simulink model "si5c_bouncing_ball_inelastic"  (R2024a)
settings: Solver=VariableStepAuto  StartTime=0.0  StopTime=10  RelTol=1e-3
values from neighbouring files (symbols this model uses):
  c = 1    [sim21_solution.m]
undefined symbols (not defined in the file or in its folder): g, h
settings Model: Creator=ocean  LastModifiedBy=ocean

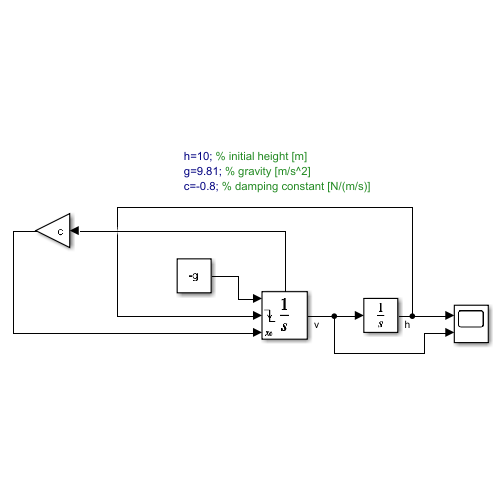
[thumbnail: Simulink's stored preview of the top-level diagram]
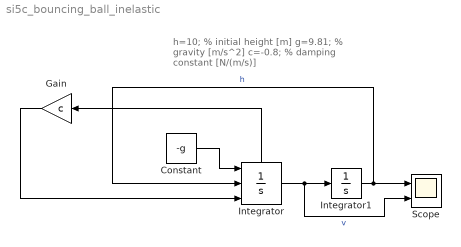
== system si5c_bouncing_ball_inelastic ==
  note: h=10; % initial height [m]
      | g=9.81; % gravity [m/s^2]
      | c=-0.8; % damping constant [N/(m/s)]
  Constant : Constant  Value=-g
  Gain : Gain  Gain=c
  Integrator : Integrator  ExternalReset=falling  InitialConditionSource=external  ShowStatePort=on
  Integrator1 : Integrator  InitialCondition=h
  Scope : Scope  NumInputPorts=2
  wires:
  Integrator/1 -> Scope/2, Integrator1/1  "v"
  Constant/1 -> Integrator/1
  Integrator1/1 -> Scope/1, Integrator/2  "h"
  Gain/1 -> Integrator/3
  Integrator/State -> Gain/1
